simulink model "qs3_interfacing"  (R2023a)
settings: Solver=ode1  StartTime=0.0  StopTime=inf  FixedStep=0.002  RelTol=1e-3
libraries: quarc_library x4
settings Model: SimulationMode=external  ExtModeTrigDuration=5000  Creator=MLevis  LastModifiedBy=Lorena Gonzalez
settings DebuggingCC: UnderspecifiedInitializationDetection=Classic  MergeDetectMultiDrivingBlocksExec=none
settings ModelReferenceCC: PropagateSignalLabelsOutOfModel=off

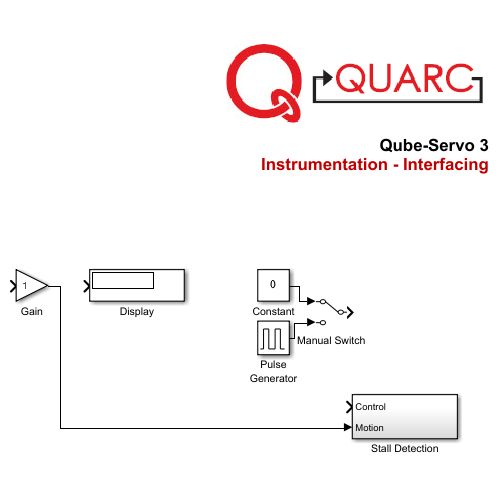
[thumbnail: Simulink's stored preview of the top-level diagram]
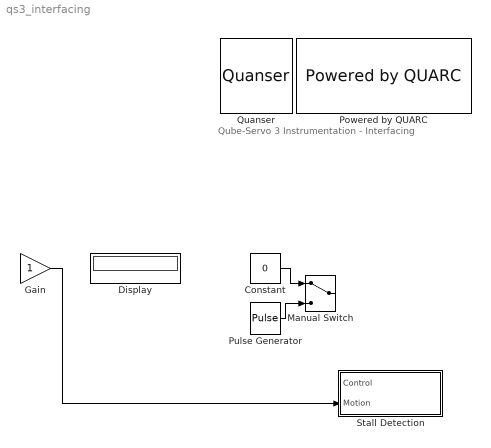
== system qs3_interfacing ==
  note: Qube-Servo 3
      | Instrumentation - Interfacing
  Constant : Constant  Value=0
  Display : Display
  Gain : Gain
  Manual Switch : ManualSwitch
  Powered by QUARC : quarc_library/Logos/Powered by QUARC
  Pulse Generator : DiscretePulseGenerator  PulseType=Time based  Amplitude=.15  Period=10  PulseWidth=20
  Quanser : quarc_library/Logos/Quanser
  Stall Detection : Subsystem
  wires:
  Gain/1 -> Stall Detection/2(Motion)
  Constant/1 -> Manual Switch/1
  Pulse Generator/1 -> Manual Switch/2

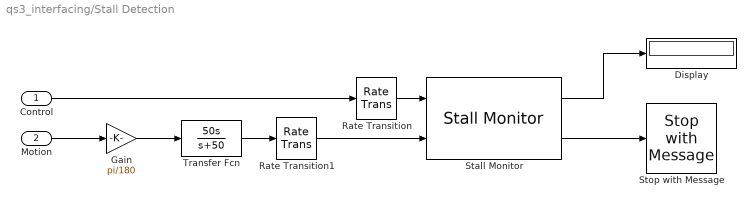
== system qs3_interfacing/Stall Detection ==
  Control : Inport
  Motion : Inport  Port=2
  Display : Display
  Gain : Gain  Gain=pi/180
  Rate Transition : RateTransition
  Rate Transition1 : RateTransition
  Stall Monitor : quarc_library/Discrete/Stall Monitor  control_threshold=1  motion_threshold=0.3  duration_s=10
      settings: SourceProductName=QUARC Targets
  Stop with Message : quarc_library/Sinks/Error Handling/Stop with Message  message_type=Fixed error message  message_icon=Error  message=Stall Detected! Please ensure that the DC motor is free to move and is functioning properly
  Transfer Fcn : TransferFcn  Numerator=[50 0]  Denominator=[1 50]
  wires:
  Control/1 -> Rate Transition/1
  Stall Monitor/2 -> Stop with Message/1
  Stall Monitor/1 -> Display/1
  Rate Transition/1 -> Stall Monitor/1
  Rate Transition1/1 -> Stall Monitor/2
  Motion/1 -> Gain/1
  Transfer Fcn/1 -> Rate Transition1/1
  Gain/1 -> Transfer Fcn/1
